simulink model "loop_shaping"  (R2015a)
settings: Solver=ode3  StartTime=0.0  StopTime=10.0  FixedStep=1/200  RelTol=1e-3
libraries: PoliArd x6
settings Model: ExtModeTrigDuration=2  Creator=GSavaia  LastModifiedBy=GSavaia
settings OptimizationCC: OptimizeModelRefInitCode=on  LifeSpan=1
settings DebuggingCC: UnderspecifiedInitializationDetection=Classic  MergeDetectMultiDrivingBlocksExec=none
settings HardwareCC: ProdLargestAtomicInteger=Long  ProdLargestAtomicFloat=Double  ProdEndianess=LittleEndian  ProdHWDeviceType=ARM Compatible->ARM Cortex
settings RTWCC: SystemTargetFile=realtime.tlc  GenerateMakefile=off  TemplateMakefile=realtime.tmf  Description=Run on Target Hardware  RTWVerbose=off
settings ERTTargetCC: CombineOutputUpdateFcns=off  ExtModeTransport=3  ExtModeMexFile=ext_serial_win32_comm_rtt  ExtModeMexArgs=0 1 9600  ERTSrcFileBannerTemplate=realtime_code_template.cgt  ERTHdrFileBannerTemplate=realtime_code_template.cgt  ERTDataSrcFileTemplate=realtime_code_template.cgt  ERTDataHdrFileTemplate=realtime_code_template.cgt  ERTCustomFileTemplate=realtime_file_process.tlc

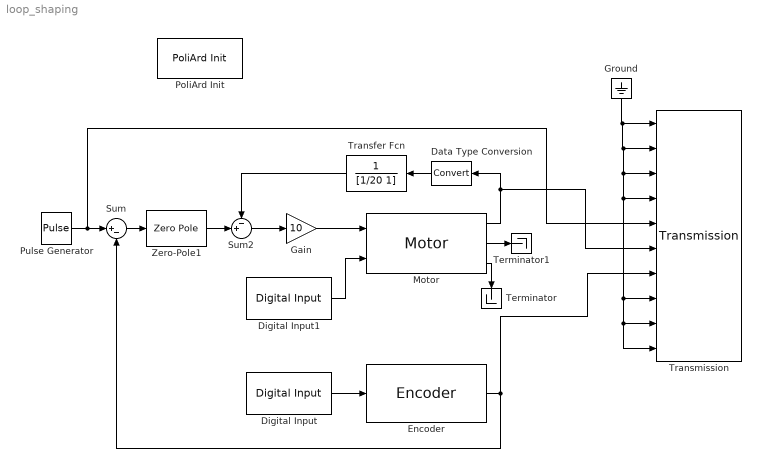
== system loop_shaping ==
  Data Type Conversion : DataTypeConversion
  Digital Input : PoliArd/Digital Input  DI_pin=2  DIsample=-1
  Digital Input1 : PoliArd/Digital Input  DI_pin=3  DIsample=-1
  Encoder : PoliArd/Encoder  EncoderID=1  dt_enc=-1
  Gain : Gain  Gain=10
  Ground : Ground
  Motor : PoliArd/Motor  MotorID=1  DC_bus_mask=12  dt_mot=-1
  PoliArd Init : PoliArd/PoliArd Init
  Pulse Generator : DiscretePulseGenerator  PulseType=Time based  Amplitude=300  Period=10  PulseWidth=50
  Sum : Sum  Inputs=|+-
  Sum2 : Sum  Inputs=-+|
  Terminator : Terminator
  Terminator1 : Terminator
  Transfer Fcn : TransferFcn  Denominator=[1/20 1]
  Transmission : PoliArd/Transmission  sample_freq=200  sig_to_send=6
  Zero-Pole1 : ZeroPole  Zeros=[-2+22i, -2-22i]  Poles=[0, -100]  Gain=-0.1
  wires:
  Digital Input/1 -> Encoder/1
  Digital Input1/1 -> Motor/2
  Gain/1 -> Motor/1
  Sum2/1 -> Gain/1
  Sum/1 -> Zero-Pole1/1
  Zero-Pole1/1 -> Sum2/2
  Encoder/1 -> Sum/2, Transmission/7
  Motor/3 -> Terminator/1
  Motor/2 -> Terminator1/1
  Pulse Generator/1 -> Transmission/5, Sum/1
  Motor/1 -> Data Type Conversion/1, Transmission/6
  Ground/1 -> Transmission/10, Transmission/9, Transmission/8, Transmission/4, Transmission/3, Transmission/2, Transmission/1
  Transfer Fcn/1 -> Sum2/1
  Data Type Conversion/1 -> Transfer Fcn/1
